simulink library "library_BCM"  (Simulink 8.2)
settings: Solver=ode45  StartTime=0.0  StopTime=10.0  RelTol=1e-3
undefined symbols (not defined in the file or in its folder): MPU_FOUR_CST, MPU_ONE_CST, MPU_THREE_CST, MPU_TWO_CST, MPU_ZERO_CST, NAMEOFTHEMODEL_SAMPLE_TIME_CST, slcm, TYP_MPU_REQUEST, TYP_MPU_REQUEST_2, TYP_MPU_STATUS, TYP_MPU_STATUS_2
libraries: Renault_Library x50, simulink x8, library_BCM x7
(part 3 of 3)

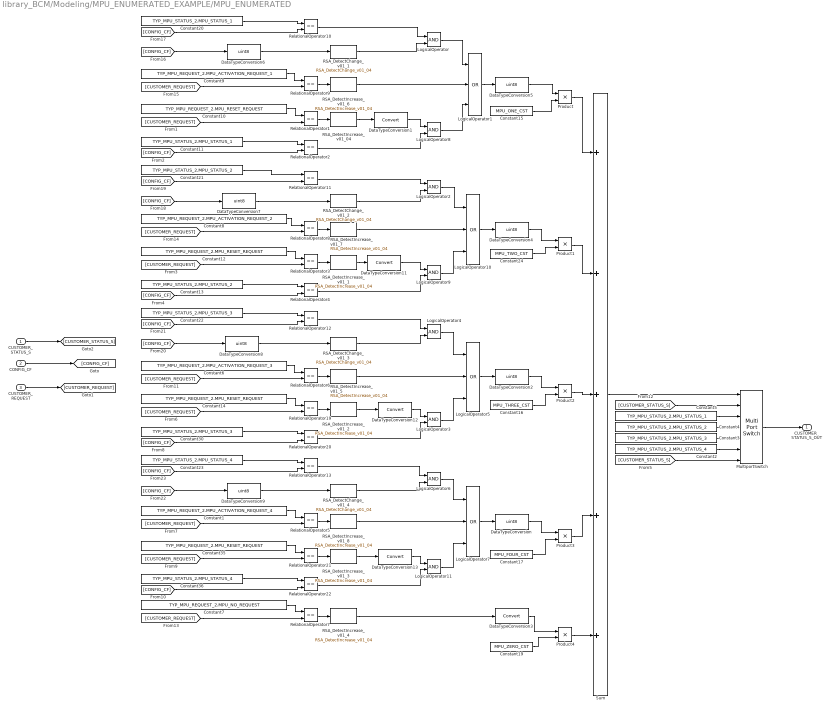
== system library_BCM/Modeling/MPU_ENUMERATED_EXAMPLE/MPU_ENUMERATED ==
  CUSTOMER_STATUS_S : Inport
      settings: AttributesFormatString=Type : %<OutDataTypeStr>
  CONFIG_CF : Inport  Port=2
      settings: AttributesFormatString=Type : %<OutDataTypeStr>
  CUSTOMER_REQUEST : Inport  Port=3
      settings: AttributesFormatString=Type : %<OutDataTypeStr>
  Constant1 : Constant  Value=TYP_MPU_REQUEST_2.MPU_ACTIVATION_REQUEST_4  OutDataTypeStr=Enum: TYP_MPU_REQUEST_2  SampleTime=-1
  Constant{10,12,14,35} (4 alike) : Constant  Value=TYP_MPU_REQUEST_2.MPU_RESET_REQUEST  OutDataTypeStr=Enum: TYP_MPU_REQUEST_2  SampleTime=-1
  Constant11 : Constant  Value=TYP_MPU_STATUS_2.MPU_STATUS_1  OutDataTypeStr=Enum: TYP_MPU_STATUS_2  SampleTime=-1
  Constant13 : Constant  Value=TYP_MPU_STATUS_2.MPU_STATUS_2  OutDataTypeStr=Enum: TYP_MPU_STATUS_2  SampleTime=-1
  Constant15 : Constant  Value=MPU_ONE_CST  OutDataTypeStr=uint8  SampleTime=-1
  Constant16 : Constant  Value=MPU_THREE_CST  OutDataTypeStr=uint8  SampleTime=-1
  Constant17 : Constant  Value=MPU_FOUR_CST  OutDataTypeStr=uint8  SampleTime=-1
  Constant19 : Constant  Value=MPU_ZERO_CST  OutDataTypeStr=uint8  SampleTime=-1
  Constant2 : Constant  Value=TYP_MPU_STATUS_2.MPU_STATUS_4  OutDataTypeStr=Enum: TYP_MPU_STATUS_2  SampleTime=-1
  Constant20 : Constant  Value=TYP_MPU_STATUS_2.MPU_STATUS_1  OutDataTypeStr=Enum: TYP_MPU_STATUS_2  SampleTime=-1
  Constant21 : Constant  Value=TYP_MPU_STATUS_2.MPU_STATUS_2  OutDataTypeStr=Enum: TYP_MPU_STATUS_2  SampleTime=-1
  Constant22 : Constant  Value=TYP_MPU_STATUS_2.MPU_STATUS_3  OutDataTypeStr=Enum: TYP_MPU_STATUS_2  SampleTime=-1
  Constant23 : Constant  Value=TYP_MPU_STATUS_2.MPU_STATUS_4  OutDataTypeStr=Enum: TYP_MPU_STATUS_2  SampleTime=-1
  Constant24 : Constant  Value=MPU_TWO_CST  OutDataTypeStr=uint8  SampleTime=-1
  Constant3 : Constant  Value=TYP_MPU_STATUS_2.MPU_STATUS_3  OutDataTypeStr=Enum: TYP_MPU_STATUS_2  SampleTime=-1
  Constant30 : Constant  Value=TYP_MPU_STATUS_2.MPU_STATUS_3  OutDataTypeStr=Enum: TYP_MPU_STATUS_2  SampleTime=-1
  Constant36 : Constant  Value=TYP_MPU_STATUS_2.MPU_STATUS_4  OutDataTypeStr=Enum: TYP_MPU_STATUS_2  SampleTime=-1
  Constant4 : Constant  Value=TYP_MPU_STATUS_2.MPU_STATUS_2  OutDataTypeStr=Enum: TYP_MPU_STATUS_2  SampleTime=-1
  Constant5 : Constant  Value=TYP_MPU_STATUS_2.MPU_STATUS_1  OutDataTypeStr=Enum: TYP_MPU_STATUS_2  SampleTime=-1
  Constant6 : Constant  Value=TYP_MPU_REQUEST_2.MPU_ACTIVATION_REQUEST_3  OutDataTypeStr=Enum: TYP_MPU_REQUEST_2  SampleTime=-1
  Constant7 : Constant  Value=TYP_MPU_REQUEST_2.MPU_NO_REQUEST  OutDataTypeStr=Enum: TYP_MPU_REQUEST_2  SampleTime=-1
  Constant8 : Constant  Value=TYP_MPU_REQUEST_2.MPU_ACTIVATION_REQUEST_2  OutDataTypeStr=Enum: TYP_MPU_REQUEST_2  SampleTime=-1
  Constant9 : Constant  Value=TYP_MPU_REQUEST_2.MPU_ACTIVATION_REQUEST_1  OutDataTypeStr=Enum: TYP_MPU_REQUEST_2  SampleTime=-1
  DataTypeConversion{,2,4..9} (8 alike) : DataTypeConversion  OutDataTypeStr=uint8  RndMeth=Zero
      settings: AttributesFormatString=Saturation:%<SaturateOnIntegerOverflow>
  DataTypeConversion{1,3,11..13} (5 alike) : DataTypeConversion  RndMeth=Zero
      settings: AttributesFormatString=Saturation:%<SaturateOnIntegerOverflow>
  LogicalOperator{,2..4,6,8..9,11} (8 alike) : Logic  OutDataTypeStr=boolean
  LogicalOperator{1,5,7,10} (4 alike) : Logic  Operator=OR  Inputs=3  OutDataTypeStr=boolean
  MultiportSwitch : MultiPortSwitch  DataPortOrder=Zero-based contiguous  Inputs=6  RndMeth=Zero  InputSameDT=on
  Product{,1..4} (5 alike) : Product  OutDataTypeStr=Inherit: Inherit via back propagation  RndMeth=Zero
  RSA_DetectChange_v01_{1..4} (4 alike) : Renault_Library/Complex blocks/Logic & Bit Operations/RSA_DetectChange_v01_04  Tag=[LIB]  chkini=off  vinit=0
      settings: AttributesFormatString=%<MaskType> : Ver : 01.04\nCompare the Input with Initial Value = %<chkini>\nInitial Value : = %<vinit>
  RSA_DetectIncrease_v01_04 : Renault_Library/Complex blocks/Logic & Bit Operations/RSA_DetectIncrease_v01_04  Tag=[LIB]  chkini=off  vinit=false
      settings: AttributesFormatString=%<MaskType> : Ver : 01.04\nCompare the Input with Initial Value = %<chkini>\nInitial Value : = %<vinit>
  RSA_DetectIncrease_v01_{1..8} (8 alike) : Renault_Library/Complex blocks/Logic & Bit Operations/RSA_DetectIncrease_v01_04  Tag=[LIB]  chkini=off  vinit=false
      settings: AttributesFormatString=%<MaskType> : Ver : 01.04\nCompare the Input with Initial Value = %<chkini>\nInitial Value : = %<vinit>
  RelationalOperator{1..13,19..22} (17 alike) : RelationalOperator  Operator===  OutDataTypeStr=boolean  InputSameDT=on
  Sum : Sum  Inputs=+++++  OutDataTypeStr=Inherit: Inherit via back propagation  RndMeth=Zero  InputSameDT=on
      settings: AttributesFormatString=Saturation:%<SaturateOnIntegerOverflow>
  CUSTOMER_STATUS_S_OUT : Outport
      settings: AttributesFormatString=Init :%<InitialOutput>
  wires:
  RelationalOperator5/1 -> RSA_DetectIncrease_v01_8/1
  LogicalOperator6/1 -> LogicalOperator7/1
  RelationalOperator13/1 -> LogicalOperator6/1
  RSA_DetectChange_v01_4/1 -> LogicalOperator6/2
  Constant23/1 -> RelationalOperator13/1
  [CONFIG_CF] -> RelationalOperator13/2
  [CONFIG_CF] -> DataTypeConversion9/1
  DataTypeConversion9/1 -> RSA_DetectChange_v01_4/1
  RelationalOperator6/1 -> RSA_DetectIncrease_v01_5/1
  LogicalOperator5/1 -> DataTypeConversion2/1
  LogicalOperator4/1 -> LogicalOperator5/1
  RelationalOperator12/1 -> LogicalOperator4/1
  RSA_DetectChange_v01_3/1 -> LogicalOperator4/2
  Constant22/1 -> RelationalOperator12/1
  [CONFIG_CF] -> RelationalOperator12/2
  [CONFIG_CF] -> DataTypeConversion8/1
  DataTypeConversion8/1 -> RSA_DetectChange_v01_3/1
  RelationalOperator8/1 -> RSA_DetectIncrease_v01_7/1
  LogicalOperator2/1 -> LogicalOperator10/1
  RelationalOperator11/1 -> LogicalOperator2/1
  RSA_DetectChange_v01_2/1 -> LogicalOperator2/2
  Constant21/1 -> RelationalOperator11/1
  [CONFIG_CF] -> RelationalOperator11/2
  [CONFIG_CF] -> DataTypeConversion7/1
  DataTypeConversion7/1 -> RSA_DetectChange_v01_2/1
  LogicalOperator1/1 -> DataTypeConversion5/1
  RelationalOperator9/1 -> RSA_DetectIncrease_v01_6/1
  LogicalOperator/1 -> LogicalOperator1/1
  RelationalOperator10/1 -> LogicalOperator/1
  RSA_DetectChange_v01_1/1 -> LogicalOperator/2
  Constant20/1 -> RelationalOperator10/1
  [CONFIG_CF] -> RelationalOperator10/2
  [CONFIG_CF] -> DataTypeConversion6/1
  DataTypeConversion6/1 -> RSA_DetectChange_v01_1/1
  Constant19/1 -> Product4/2
  Constant17/1 -> Product3/2
  Constant16/1 -> Product2/2
  Constant24/1 -> Product1/2
  Constant15/1 -> Product/2
  Product/1 -> Sum/1
  Product1/1 -> Sum/2
  Product2/1 -> Sum/3
  Product3/1 -> Sum/4
  Product4/1 -> Sum/5
  DataTypeConversion5/1 -> Product/1
  Constant9/1 -> RelationalOperator9/1
  [CUSTOMER_REQUEST] -> RelationalOperator9/2
  DataTypeConversion4/1 -> Product1/1
  Constant8/1 -> RelationalOperator8/1
  [CUSTOMER_REQUEST] -> RelationalOperator8/2
  DataTypeConversion3/1 -> Product4/1
  Constant7/1 -> RelationalOperator7/1
  [CUSTOMER_REQUEST] -> RelationalOperator7/2
  DataTypeConversion2/1 -> Product2/1
  DataTypeConversion/1 -> Product3/1
  Sum/1 -> MultiportSwitch/1
  Constant6/1 -> RelationalOperator6/1
  [CUSTOMER_REQUEST] -> RelationalOperator6/2
  Constant1/1 -> RelationalOperator5/1
  [CUSTOMER_REQUEST] -> RelationalOperator5/2
  [CUSTOMER_STATUS_S] -> MultiportSwitch/7
  MultiportSwitch/1 -> CUSTOMER_STATUS_S_OUT/1
  CONFIG_CF/1 -> [CONFIG_CF]
  CUSTOMER_REQUEST/1 -> [CUSTOMER_REQUEST]
  CUSTOMER_STATUS_S/1 -> [CUSTOMER_STATUS_S]
  RelationalOperator7/1 -> RSA_DetectIncrease_v01_4/1
  RelationalOperator1/1 -> RSA_DetectIncrease_v01_04/1
  Constant10/1 -> RelationalOperator1/1
  [CUSTOMER_REQUEST] -> RelationalOperator1/2
  RSA_DetectIncrease_v01_04/1 -> DataTypeConversion1/1
  RelationalOperator2/1 -> LogicalOperator8/2
  Constant11/1 -> RelationalOperator2/1
  [CONFIG_CF] -> RelationalOperator2/2
  DataTypeConversion1/1 -> LogicalOperator8/1
  LogicalOperator8/1 -> LogicalOperator1/3
  RelationalOperator3/1 -> RSA_DetectIncrease_v01_1/1
  Constant12/1 -> RelationalOperator3/1
  [CUSTOMER_REQUEST] -> RelationalOperator3/2
  RSA_DetectIncrease_v01_1/1 -> DataTypeConversion11/1
  RelationalOperator4/1 -> LogicalOperator9/2
  Constant13/1 -> RelationalOperator4/1
  [CONFIG_CF] -> RelationalOperator4/2
  DataTypeConversion11/1 -> LogicalOperator9/1
  LogicalOperator9/1 -> LogicalOperator10/3
  LogicalOperator10/1 -> DataTypeConversion4/1
  RelationalOperator19/1 -> RSA_DetectIncrease_v01_2/1
  Constant14/1 -> RelationalOperator19/1
  [CUSTOMER_REQUEST] -> RelationalOperator19/2
  RSA_DetectIncrease_v01_2/1 -> DataTypeConversion12/1
  RelationalOperator20/1 -> LogicalOperator3/2
  Constant30/1 -> RelationalOperator20/1
  [CONFIG_CF] -> RelationalOperator20/2
  DataTypeConversion12/1 -> LogicalOperator3/1
  LogicalOperator3/1 -> LogicalOperator5/3
  RelationalOperator21/1 -> RSA_DetectIncrease_v01_3/1
  Constant35/1 -> RelationalOperator21/1
  [CUSTOMER_REQUEST] -> RelationalOperator21/2
  RSA_DetectIncrease_v01_3/1 -> DataTypeConversion13/1
  RelationalOperator22/1 -> LogicalOperator11/2
  Constant36/1 -> RelationalOperator22/1
  [CONFIG_CF] -> RelationalOperator22/2
  DataTypeConversion13/1 -> LogicalOperator11/1
  LogicalOperator7/1 -> DataTypeConversion/1
  LogicalOperator11/1 -> LogicalOperator7/3
  RSA_DetectIncrease_v01_4/1 -> DataTypeConversion3/1
  RSA_DetectIncrease_v01_5/1 -> LogicalOperator5/2
  RSA_DetectIncrease_v01_6/1 -> LogicalOperator1/2
  RSA_DetectIncrease_v01_7/1 -> LogicalOperator10/2
  RSA_DetectIncrease_v01_8/1 -> LogicalOperator7/2
  [CUSTOMER_STATUS_S] -> MultiportSwitch/2
  Constant2/1 -> MultiportSwitch/6
  Constant5/1 -> MultiportSwitch/3
  Constant3/1 -> MultiportSwitch/5
  Constant4/1 -> MultiportSwitch/4

== system library_BCM/Validation/EEPROM/DataStoreRead ==
  Data Store Read : DataStoreRead  DataStoreName=EEPROM_S
  EEPROM_S_N : Outport
  wires:
  Data Store Read/1 -> EEPROM_S_N/1

== system library_BCM/Validation/EEPROM/DataStoreWrite ==
  EEPROM_S : Inport
  EEPROM_S_OUT : Inport  Port=2
  ECU_RESET : Inport  Port=3
  Detect Change : simulink/Logic and Bit Operations/Detect Change  vinit=0  InputProcessing=Inherited  OutDataTypeStr=boolean
  Detect Change2 : simulink/Logic and Bit Operations/Detect Change  vinit=0  InputProcessing=Inherited  OutDataTypeStr=boolean
  Detect Change4 : simulink/Logic and Bit Operations/Detect Change  vinit=0  InputProcessing=Inherited  OutDataTypeStr=boolean
  Logical Operator : Logic  AllPortsSameDT=off  OutDataTypeStr=boolean
  Logical Operator1 : Logic  Operator=NOT  AllPortsSameDT=off  OutDataTypeStr=boolean
  Subsystem : Subsystem
  Switch : Switch  Criteria=u2 ~= 0
  Switch1 : Switch  Criteria=u2 ~= 0
  Switch4 : Switch  Criteria=u2 ~= 0
  Unit Delay : UnitDelay  SampleTime=-1
  wires:
  EEPROM_S/1 -> Detect Change/1, Switch/1
  Detect Change/1 -> Switch/2
  Detect Change2/1 -> Logical Operator/1
  Logical Operator/1 -> Switch4/2
  Switch4/1 -> Switch1/3, Switch/3
  Switch/1 -> Switch1/1, Subsystem/1(In), Detect Change4/1
  Unit Delay/1 -> Switch4/3
  EEPROM_S_OUT/1 -> Detect Change2/1, Switch4/1
  Detect Change4/1 -> Subsystem/Enable
  ECU_RESET/1 -> [RESET], Logical Operator/2
  Logical Operator1/1 -> Switch1/2
  [RESET] -> Logical Operator1/1
  Switch1/1 -> Unit Delay/1

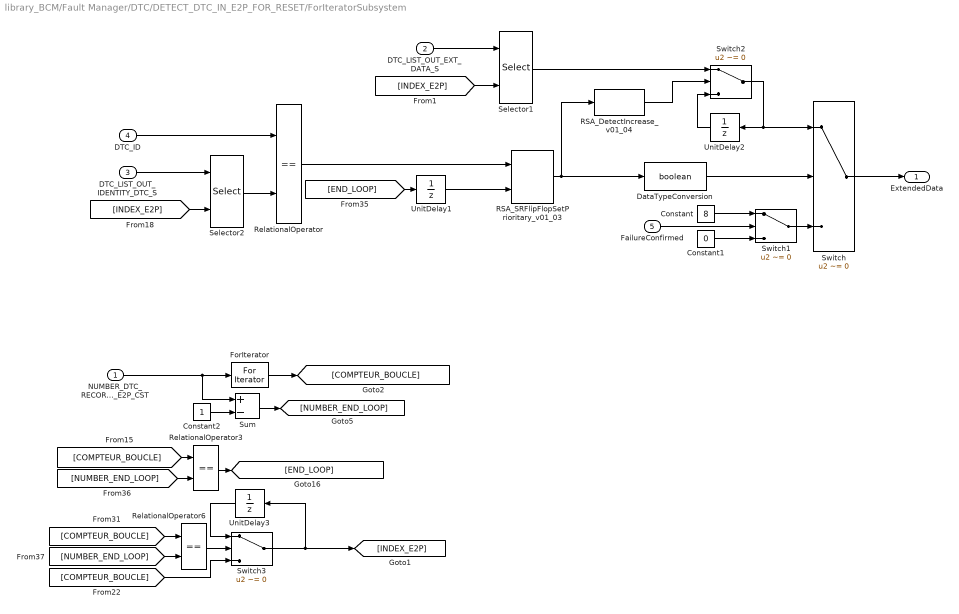
== system library_BCM/Fault Manager/DTC/DETECT_DTC_IN_E2P_FOR_RESET/ForIteratorSubsystem ==
  NUMBER_DTC_RECORD_IN_E2P_CST : Inport  OutDataTypeStr=uint32
      settings: AttributesFormatString=Type : %<OutDataTypeStr>
  DTC_LIST_OUT_EXT_DATA_S : Inport  Port=2  OutDataTypeStr=uint32
      settings: AttributesFormatString=Type : %<OutDataTypeStr>
  DTC_LIST_OUT_IDENTITY_DTC_S : Inport  Port=3  OutDataTypeStr=uint32
      settings: AttributesFormatString=Type : %<OutDataTypeStr>
  DTC_ID : Inport  Port=4  OutDataTypeStr=uint32
      settings: AttributesFormatString=Type : %<OutDataTypeStr>
  FailureConfirmed : Inport  Port=5  OutDataTypeStr=boolean
      settings: AttributesFormatString=Type : %<OutDataTypeStr>
  Constant : Constant  Value=8  OutDataTypeStr=uint32  SampleTime=-1
  Constant1 : Constant  Value=0  OutDataTypeStr=uint32  SampleTime=-1
  Constant2 : Constant  OutDataTypeStr=uint32  SampleTime=-1
  DataTypeConversion : DataTypeConversion  OutDataTypeStr=boolean  RndMeth=Zero
      settings: AttributesFormatString=Saturation:%<SaturateOnIntegerOverflow>
  ForIterator : ForIterator  IterationSource=external  IndexMode=Zero-based
  RSA_DetectIncrease_v01_04 : Renault_Library/Complex blocks/Logic & Bit Operations/RSA_DetectIncrease_v01_04  Tag=[LIB]  chkini=on  vinit=0
      settings: AttributesFormatString=%<MaskType> : Ver : 01.04\nCompare the Input with Initial Value = %<chkini>\nInitial Value : = %<vinit>
  RSA_SRFlipFlopSetPrioritary_v01_03 : Renault_Library/Complex blocks/Flip-Flop/RSA_SRFlipFlopSetPrioritary_v01_03  Tag=[LIB]  init=false
      settings: AttributesFormatString=%<MaskType> : Ver : 01.03\n<init=%<init>>
  RelationalOperator : RelationalOperator  Operator===  OutDataTypeStr=boolean  InputSameDT=on
  RelationalOperator3 : RelationalOperator  Operator===  OutDataTypeStr=boolean  InputSameDT=on
  RelationalOperator6 : RelationalOperator  Operator===  OutDataTypeStr=boolean  InputSameDT=on
  Selector1 : Selector  IndexMode=Zero-based  IndexOptions=Index vector (port)  Indices=[1 3]  OutputSizes=1
  Selector2 : Selector  IndexMode=Zero-based  IndexOptions=Index vector (port)  Indices=[1 3]  OutputSizes=1
  Sum : Sum  Inputs=+-  AccumDataTypeStr=uint32  OutDataTypeStr=Inherit: Inherit via back propagation  RndMeth=Zero  InputSameDT=on
      settings: AttributesFormatString=Saturation:%<SaturateOnIntegerOverflow>
  Switch{,1..3} (4 alike) : Switch  Criteria=u2 ~= 0  RndMeth=Zero  InputSameDT=on
      settings: AttributesFormatString=Criteria=%<Criteria>
  UnitDelay1 : UnitDelay  SampleTime=-1
      settings: AttributesFormatString=IC = %<X0>
  UnitDelay2 : UnitDelay  SampleTime=-1
      settings: AttributesFormatString=IC = %<X0>
  UnitDelay3 : UnitDelay  SampleTime=-1
      settings: AttributesFormatString=IC = %<X0>
  ExtendedData : Outport  OutDataTypeStr=uint32  InitialOutput=0
      settings: CopyFcn=if exist('tl_check_ports','file'), tl_check_ports(gcbh); end  NameChangeFcn=if exist('tl_check_ports','file'), tl_check_ports(gcbh); end
  wires:
  Constant1/1 -> Switch1/3
  Constant/1 -> Switch1/1
  Switch1/1 -> Switch/3
  FailureConfirmed/1 -> Switch1/2
  Switch/1 -> ExtendedData/1
  [INDEX_E2P] -> Selector1/2
  DTC_LIST_OUT_EXT_DATA_S/1 -> Selector1/1
  Selector2/1 -> RelationalOperator/2
  [INDEX_E2P] -> Selector2/2
  NUMBER_DTC_RECORD_IN_E2P_CST/1 -> ForIterator/1, Sum/1
  ForIterator/1 -> [COMPTEUR_BOUCLE]
  DTC_LIST_OUT_IDENTITY_DTC_S/1 -> Selector2/1
  DTC_ID/1 -> RelationalOperator/1
  [NUMBER_END_LOOP] -> RelationalOperator6/2
  UnitDelay3/1 -> Switch3/1
  [COMPTEUR_BOUCLE] -> Switch3/3
  RelationalOperator6/1 -> Switch3/2
  [COMPTEUR_BOUCLE] -> RelationalOperator6/1
  Switch3/1 -> UnitDelay3/1, [INDEX_E2P]
  [NUMBER_END_LOOP] -> RelationalOperator3/2
  RelationalOperator3/1 -> [END_LOOP]
  [COMPTEUR_BOUCLE] -> RelationalOperator3/1
  Constant2/1 -> Sum/2
  Sum/1 -> [NUMBER_END_LOOP]
  RelationalOperator/1 -> RSA_SRFlipFlopSetPrioritary_v01_03/1
  RSA_SRFlipFlopSetPrioritary_v01_03/1 -> DataTypeConversion/1, RSA_DetectIncrease_v01_04/1
  UnitDelay2/1 -> Switch2/3
  RSA_DetectIncrease_v01_04/1 -> Switch2/2
  [END_LOOP] -> UnitDelay1/1
  Switch2/1 -> UnitDelay2/1, Switch/1
  Selector1/1 -> Switch2/1
  UnitDelay1/1 -> RSA_SRFlipFlopSetPrioritary_v01_03/2
  DataTypeConversion/1 -> Switch/2

== system library_BCM/Fault Manager/DTC/DETECT_DTC_IN_E2P_FOR_RESET/TO_ADD_1_CALCUL_IN_LOOP ==
  NUMBER_DTC_RECORD_IN_E2P_CST : Inport  OutDataTypeStr=uint32
      settings: AttributesFormatString=Type : %<OutDataTypeStr>
  Constant : Constant  OutDataTypeStr=Inherit: Inherit via back propagation  SampleTime=-1
  Sum : Sum  OutDataTypeStr=Inherit: Inherit via back propagation  RndMeth=Zero  InputSameDT=on
      settings: AttributesFormatString=Saturation: %<SaturateOnIntegerOverflow>
  NB_DTC_RECORD_IN_E2P_CST_EXT : Outport  OutDataTypeStr=uint32
  wires:
  NUMBER_DTC_RECORD_IN_E2P_CST/1 -> Sum/1
  Constant/1 -> Sum/2
  Sum/1 -> NB_DTC_RECORD_IN_E2P_CST_EXT/1

== system library_BCM/Fault Manager/DTC/ExtendedData_Calcul/BitwiseLogicalOperator3 ==
  u : Inport
  shift : ArithShift  BitShiftNumber=nBitShiftRight  BinPtShiftNumber=nBinPtShiftRight
  y : Outport
  wires:
  u/1 -> shift/1
  shift/1 -> y/1

== system library_BCM/Fault Manager/DTC/ExtendedData_Calcul/BitwiseLogicalOperator6 ==
  u : Inport
  shift : ArithShift  BitShiftNumber=nBitShiftRight  BinPtShiftNumber=nBinPtShiftRight
  y : Outport
  wires:
  shift/1 -> y/1
  u/1 -> shift/1

== system library_BCM/MIL Full Matlab/Scheduling/Lib_Trigger/Trigger ==
  In1 : Inport
      settings: AttributesFormatString=Type : %<OutDataTypeStr>
  RSA_Bias1 : Subsystem  Tag=[LIB]  mask(RSA_Bias){u=1, DoSatur=off}
      mask prompts: u "Bias:"; DoSatur "Saturate on integer overflow"
      mask help:
      | Add bias to input,Y = U + Bias.
      |
      | Version : 01.00
      mask init:
      | blkH = gcbh;
      | blkName = getfullname(blkH);
      mask Display: %fprintf('u + %d', u)
  RSA_Bias2 : Subsystem  Tag=[LIB]  mask(RSA_Bias){u=-1, DoSatur=off}
      mask prompts: u "Bias:"; DoSatur "Saturate on integer overflow"
      mask help:
      | Add bias to input,Y = U + Bias.
      |
      | Version : 01.00
      mask init:
      | blkH = gcbh;
      | blkName = getfullname(blkH);
      mask Display: %fprintf('u + %d', u)
  RSA_DetectChange : Renault_Library/Complex blocks/Logic & Bit Operations/RSA_DetectChange  Tag=[LIB]  vinit=0
  RSA_DivisionByZeroWithSaturation1 : Subsystem  Tag=[LIB]  mask(RSA_DivisionByZeroWithSaturation){}
      mask help:
      | The given two inputs 'In1' and 'In2' are divided and the output 'Out1' is obtained. If the 'In2' is zero then output 'Out1' retain the input 'In1'.
      |
      | Version : 01.00
      mask Display:
      | % plot([4 12],[32 40])
      | % plot([4 12],[40 32])
      | %
      | % plot([4 12],[12 12])
      | %
      | % plot([8 8],[16 16])
      | % plot([7 9],[15 15])
      | % plot([8 8],[14 14])
      | %
      | % plot([8 8],[10 10])
      | % plot([7 9],[9 9])
      | % plot([8 8],[8 8])
  UnitDelay2 : UnitDelay  SampleTime=-1
  Out1 : Outport
      settings: AttributesFormatString=Type : %<OutDataTypeStr>\nInit :%<InitialOutput>
  wires:
  RSA_Bias1/1(Out1) -> UnitDelay2/1, RSA_Bias2/1(In1)
  UnitDelay2/1 -> RSA_Bias1/1(In1)
  RSA_Bias2/1(Out1) -> RSA_DivisionByZeroWithSaturation1/1(In1)
  RSA_DivisionByZeroWithSaturation1/1(Out1) -> RSA_DetectChange/1
  RSA_DetectChange/1 -> Out1/1
  In1/1 -> RSA_DivisionByZeroWithSaturation1/2(In2)

== system library_BCM/MIL Full Matlab/Scheduling0/Lib_Trigger/Trigger ==
  In1 : Inport
      settings: AttributesFormatString=Type : %<OutDataTypeStr>
  RSA_Bias1 : Subsystem  Tag=[LIB]  mask(RSA_Bias){u=1, DoSatur=off}
      mask prompts: u "Bias:"; DoSatur "Saturate on integer overflow"
      mask help:
      | Add bias to input,Y = U + Bias.
      |
      | Version : 01.00
      mask init:
      | blkH = gcbh;
      | blkName = getfullname(blkH);
      mask Display: %fprintf('u + %d', u)
  RSA_Bias2 : Subsystem  Tag=[LIB]  mask(RSA_Bias){u=-1, DoSatur=off}
      mask prompts: u "Bias:"; DoSatur "Saturate on integer overflow"
      mask help:
      | Add bias to input,Y = U + Bias.
      |
      | Version : 01.00
      mask init:
      | blkH = gcbh;
      | blkName = getfullname(blkH);
      mask Display: %fprintf('u + %d', u)
  RSA_DetectChange : Renault_Library/Complex blocks/Logic & Bit Operations/RSA_DetectChange  Tag=[LIB]  vinit=0
  RSA_DivisionByZeroWithSaturation1 : Subsystem  Tag=[LIB]  mask(RSA_DivisionByZeroWithSaturation){}
      mask help:
      | The given two inputs 'In1' and 'In2' are divided and the output 'Out1' is obtained. If the 'In2' is zero then output 'Out1' retain the input 'In1'.
      |
      | Version : 01.00
      mask Display:
      | % plot([4 12],[32 40])
      | % plot([4 12],[40 32])
      | %
      | % plot([4 12],[12 12])
      | %
      | % plot([8 8],[16 16])
      | % plot([7 9],[15 15])
      | % plot([8 8],[14 14])
      | %
      | % plot([8 8],[10 10])
      | % plot([7 9],[9 9])
      | % plot([8 8],[8 8])
  UnitDelay2 : UnitDelay  SampleTime=-1
  Out1 : Outport
      settings: AttributesFormatString=Type : %<OutDataTypeStr>\nInit :%<InitialOutput>
  wires:
  In1/1 -> RSA_DivisionByZeroWithSaturation1/2(In2)
  RSA_DetectChange/1 -> Out1/1
  RSA_DivisionByZeroWithSaturation1/1(Out1) -> RSA_DetectChange/1
  RSA_Bias2/1(Out1) -> RSA_DivisionByZeroWithSaturation1/1(In1)
  UnitDelay2/1 -> RSA_Bias1/1(In1)
  RSA_Bias1/1(Out1) -> RSA_Bias2/1(In1), UnitDelay2/1

== system library_BCM/Validation/EEPROM/DataStoreWrite/Subsystem ==
  In : Inport
  Enable : EnablePort  StatesWhenEnabling=reset
  Data Store Write : DataStoreWrite  DataStoreName=EEPROM_S
  wires:
  In/1 -> Data Store Write/1

== system library_BCM/MIL Full Matlab/Scheduling/Lib_Trigger/Trigger/RSA_Bias1 ==
  In1 : Inport
      settings: AttributesFormatString=Type : %<OutDataType>\nScaling : %<OutScaling>
  Add : Sum  OutDataTypeStr=Inherit: Inherit via back propagation  RndMeth=Zero  InputSameDT=on
  Constant1 : Constant  Value=u  OutDataTypeStr=Inherit: Inherit via back propagation  SampleTime=-1
  Out1 : Outport
      settings: AttributesFormatString=Type : %<OutDataType>\nScaling : %<OutScaling>\nInit :%<InitialOutput>
  wires:
  Constant1/1 -> Add/2
  In1/1 -> Add/1
  Add/1 -> Out1/1

== system library_BCM/MIL Full Matlab/Scheduling/Lib_Trigger/Trigger/RSA_Bias2 ==
  In1 : Inport
      settings: AttributesFormatString=Type : %<OutDataType>\nScaling : %<OutScaling>
  Add : Sum  OutDataTypeStr=Inherit: Inherit via back propagation  RndMeth=Zero  InputSameDT=on
  Constant1 : Constant  Value=u  OutDataTypeStr=Inherit: Inherit via back propagation  SampleTime=-1
  Out1 : Outport
      settings: AttributesFormatString=Type : %<OutDataType>\nScaling : %<OutScaling>\nInit :%<InitialOutput>
  wires:
  Add/1 -> Out1/1
  In1/1 -> Add/1
  Constant1/1 -> Add/2

== system library_BCM/MIL Full Matlab/Scheduling/Lib_Trigger/Trigger/RSA_DivisionByZeroWithSaturation1 ==
  In1 : Inport
      settings: AttributesFormatString=Type : %<OutDataType>\nScaling : %<OutScaling>
  In2 : Inport  Port=2
      settings: AttributesFormatString=Type : %<OutDataType>\nScaling : %<OutScaling>
  Product2 : Product  Inputs=*/  OutDataTypeStr=Inherit: Inherit via back propagation  RndMeth=Zero  InputSameDT=on
  RSA_CompareToZero : Subsystem  Tag=[LIB]  mask(RSA_CompareToZero){relop===, LogicOutDataTypeMode=boolean, ZeroCross=on}
      mask prompts: relop "Operator:"; LogicOutDataTypeMode "Output data type mode:"; ZeroCross "Enable zero-crossing detection"
      mask help:
      | Output of the block will be zero when the signal is less than or equal to zero otherwise it will be one.
      |
      | Version : 01.00
      mask init:
      | blkName = gcb;
      mask TypeOptions relop: == | ~= | < | <= | >= | >
      mask TypeOptions LogicOutDataTypeMode: uint8 | boolean
      mask Display: disp([relop,' 0'])
  Switch1 : Switch  Criteria=u2 ~= 0  RndMeth=Zero  SaturateOnIntegerOverflow=on  InputSameDT=on
  const1 : Constant  OutDataTypeStr=Inherit: Inherit via back propagation  SampleTime=-1
  Out1 : Outport
      settings: AttributesFormatString=Type : %<OutDataType>\nScaling : %<OutScaling>\nInit :%<InitialOutput>
  wires:
  In1/1 -> Product2/1
  Product2/1 -> Out1/1
  const1/1 -> Switch1/1
  Switch1/1 -> Product2/2
  RSA_CompareToZero/1(y) -> Switch1/2
  In2/1 -> Switch1/3, RSA_CompareToZero/1(u)

== system library_BCM/MIL Full Matlab/Scheduling0/Lib_Trigger/Trigger/RSA_Bias1 ==
  In1 : Inport
      settings: AttributesFormatString=Type : %<OutDataType>\nScaling : %<OutScaling>
  Add : Sum  OutDataTypeStr=Inherit: Inherit via back propagation  RndMeth=Zero  InputSameDT=on
  Constant1 : Constant  Value=u  OutDataTypeStr=Inherit: Inherit via back propagation  SampleTime=-1
  Out1 : Outport
      settings: AttributesFormatString=Type : %<OutDataType>\nScaling : %<OutScaling>\nInit :%<InitialOutput>
  wires:
  Add/1 -> Out1/1
  In1/1 -> Add/1
  Constant1/1 -> Add/2

== system library_BCM/MIL Full Matlab/Scheduling0/Lib_Trigger/Trigger/RSA_Bias2 ==
  In1 : Inport
      settings: AttributesFormatString=Type : %<OutDataType>\nScaling : %<OutScaling>
  Add : Sum  OutDataTypeStr=Inherit: Inherit via back propagation  RndMeth=Zero  InputSameDT=on
  Constant1 : Constant  Value=u  OutDataTypeStr=Inherit: Inherit via back propagation  SampleTime=-1
  Out1 : Outport
      settings: AttributesFormatString=Type : %<OutDataType>\nScaling : %<OutScaling>\nInit :%<InitialOutput>
  wires:
  Constant1/1 -> Add/2
  In1/1 -> Add/1
  Add/1 -> Out1/1

== system library_BCM/MIL Full Matlab/Scheduling0/Lib_Trigger/Trigger/RSA_DivisionByZeroWithSaturation1 ==
  In1 : Inport
      settings: AttributesFormatString=Type : %<OutDataType>\nScaling : %<OutScaling>
  In2 : Inport  Port=2
      settings: AttributesFormatString=Type : %<OutDataType>\nScaling : %<OutScaling>
  Product2 : Product  Inputs=*/  OutDataTypeStr=Inherit: Inherit via back propagation  RndMeth=Zero  InputSameDT=on
  RSA_CompareToZero : Subsystem  Tag=[LIB]  mask(RSA_CompareToZero){relop===, LogicOutDataTypeMode=boolean, ZeroCross=on}
      mask prompts: relop "Operator:"; LogicOutDataTypeMode "Output data type mode:"; ZeroCross "Enable zero-crossing detection"
      mask help:
      | Output of the block will be zero when the signal is less than or equal to zero otherwise it will be one.
      |
      | Version : 01.00
      mask init:
      | blkName = gcb;
      mask TypeOptions relop: == | ~= | < | <= | >= | >
      mask TypeOptions LogicOutDataTypeMode: uint8 | boolean
      mask Display: disp([relop,' 0'])
  Switch1 : Switch  Criteria=u2 ~= 0  RndMeth=Zero  SaturateOnIntegerOverflow=on  InputSameDT=on
  const1 : Constant  OutDataTypeStr=Inherit: Inherit via back propagation  SampleTime=-1
  Out1 : Outport
      settings: AttributesFormatString=Type : %<OutDataType>\nScaling : %<OutScaling>\nInit :%<InitialOutput>
  wires:
  In2/1 -> RSA_CompareToZero/1(u), Switch1/3
  RSA_CompareToZero/1(y) -> Switch1/2
  Switch1/1 -> Product2/2
  const1/1 -> Switch1/1
  Product2/1 -> Out1/1
  In1/1 -> Product2/1

== system library_BCM/MIL Full Matlab/Scheduling/Lib_Trigger/Trigger/RSA_DivisionByZeroWithSaturation1/RSA_CompareToZero ==
  u : Inport
      settings: AttributesFormatString=Type : %<OutDataType>\nScaling : %<OutScaling>
  Compare : RelationalOperator  Operator===  OutDataTypeStr=boolean  InputSameDT=on
  Constant : Constant  DisableCoverage=on  Value=0  OutDataTypeStr=Inherit: Inherit via back propagation  SampleTime=-1  PreserveConstantTs=on
  y : Outport
      settings: AttributesFormatString=Type : %<OutDataType>\nScaling : %<OutScaling>\nInit :%<InitialOutput>
  wires:
  Constant/1 -> Compare/2
  u/1 -> Compare/1
  Compare/1 -> y/1

== system library_BCM/MIL Full Matlab/Scheduling0/Lib_Trigger/Trigger/RSA_DivisionByZeroWithSaturation1/RSA_CompareToZero ==
  u : Inport
      settings: AttributesFormatString=Type : %<OutDataType>\nScaling : %<OutScaling>
  Compare : RelationalOperator  Operator===  OutDataTypeStr=boolean  InputSameDT=on
  Constant : Constant  DisableCoverage=on  Value=0  OutDataTypeStr=Inherit: Inherit via back propagation  SampleTime=-1  PreserveConstantTs=on
  y : Outport
      settings: AttributesFormatString=Type : %<OutDataType>\nScaling : %<OutScaling>\nInit :%<InitialOutput>
  wires:
  Compare/1 -> y/1
  u/1 -> Compare/1
  Constant/1 -> Compare/2

== stateflow chart Validation/EEPROM_OLD/Chart ==
  state A
  (default) -> A : {
      | x=1;
      | }
  A -> A [order 1] : [hasChanged(WRITE)]
      | {
      | x=2;
      | }
  A -> A [order 2] : [hasChanged(READ)]
      | {
      | x=1;
      | }
  data: READ input double; WRITE input double; x output double

== stateflow chart Fault Manager/EEPROM_SNAPSHOT/EEPROM_FCT/EEPROM_chart ==
  note: /*effacement de l'indice du DTC ecrit */
  note: /*mise à jour SNAPSHOT*/
  note: /*i_IDENTITYFULL = 0 ==> init
      | i_IDENTITYFULL = 1==> new DTC already saved in EEPROM
      | i_IDENTITYFULL = 2 ==> new DTC is not saved in EEPROM and empty case is available
      | i_IDENTITYFULL =3 ==> new DTC is not saved in EEPROM and empty case is not available*/
  (default) -> (junction 50) : /* boucle recupération index TCONF montés */
      | {i_RAM=0;
      | i_TCONF=0;
      | DTC_LIST_OUT_OCCUR_CNT_S_INT=DTC_LIST_OUT_OCCUR_CNT_S;
      | DTC_LIST_OUT_EXT_DATA_S_INT=DTC_LIST_OUT_EXT_DATA_S;
      | DTC_LIST_OUT_IDENTITY_DTC_S_INT=DTC_LIST_OUT_IDENTITY_DTC_S;
      | DTC_LIST_OUT_SNAPSHOT_S_INT=DTC_LIST_OUT_SNAPSHOT_S;
      | NB_PRESENT_DTC_S_INT=NB_PRESENT_DTC_S;
      | NUMBER_TCONF_TO_UPDATE=NUMBER_TCONF_UP;}
  (junction 51) -> (junction 50) [order 1] : [i_RAM<NUMBER_DTC_RECORD_IN_RAM]
  (junction 50) -> (junction 51) [order 1] : [TCONF_CHANGED[i_RAM]==1]
      | {TCONF_CHANGED_SIMPLIFIED[i_TCONF]=i_RAM;
      | i_TCONF=i_TCONF+1;
      | i_RAM=i_RAM+1;}
  (junction 50) -> (junction 51) [order 2] : {i_RAM=i_RAM+1;}
  (junction 51) -> (junction 52) [order 2] : /* boucle vérification déjà présent */
      | {i_TCONF=0;
      | i_SNAPSHOT=0;
      | i_EEPROM=0;
      | i_IDENTITYFULL=0;}
  (junction 53) -> (junction 54) [order 1] : [(((STATUS_TABLE[TCONF_CHANGED_SIMPLIFIED[i_TCONF]])&0xFFFFFFF0)>>4)!=0x0FFFFFFF]
      | {
      | DTC_LIST_OUT_EXT_DATA_S_INT[i_EEPROM]=STATUS_TABLE[TCONF_CHANGED_SIMPLIFIED[i_TCONF]];
      | }
  (junction 52) -> (junction 53) [order 2] : [DTC_ID[TCONF_CHANGED_SIMPLIFIED[i_TCONF]]==DTC_LIST_OUT_IDENTITY_DTC_S_INT[i_EEPROM]]
      | {
      | DTC_LIST_OUT_IDENTITY_DTC_S_INT[i_EEPROM]=DTC_ID[TCONF_CHANGED_SIMPLIFIED[i_TCONF]];
      | i_TCONF_TEMP=i_TCONF;
      | NUMBER_TCONF_TO_UPDATE=NUMBER_TCONF_TO_UPDATE-1;
      | i_IDENTITYFULL=1;
      | }
  (junction 52) -> (junction 61) [order 1] : /*pas de DTC à cet index */
      | [DTC_ID[TCONF_CHANGED_SIMPLIFIED[i_TCONF]]==0]
  (junction 53) -> (junction 54) [order 2]
  (junction 54) -> (junction 60) [order 1] : [DTC_LIST_OUT_OCCUR_CNT_S_INT[i_EEPROM]==255]
  (junction 56) -> (junction 52) [order 1] : [i_TCONF<NUMBER_TCONF_TO_UPDATE]
  (junction 52) -> (junction 57) [order 3] : {i_EEPROM=i_EEPROM+1;}
  (junction 54) -> (junction 60) [order 2] : {DTC_LIST_OUT_OCCUR_CNT_S_INT[i_EEPROM]=DTC_LIST_OUT_OCCUR_CNT_S_INT[i_EEPROM]+1;}
  (junction 55) -> (junction 58) [order 1] : [i_TCONF_TEMP<NUMBER_TCONF_TO_UPDATE-1]
      | {i_TCONF_TEMP=i_TCONF_TEMP+1;}
  (junction 59) -> (junction 60) [order 1] : [i_SNAPSHOT<SNAPSHOT_MAX_LENGHT-1]
      | {i_SNAPSHOT=i_SNAPSHOT+1;}
  (junction 55) -> (junction 57) [order 3] : {i_EEPROM=0;}
  (junction 57) -> (junction 56) [order 2] : {i_TCONF=i_TCONF+1;
      | i_EEPROM=0;}
  (junction 59) -> (junction 58) [order 2] : [i_IDENTITYFULL!=3]{i_SNAPSHOT=0;}
  (junction 56) -> (junction 61) [order 2]
  (junction 60) -> (junction 59) [order 3] : {DTC_LIST_OUT_SNAPSHOT_S_INT[i_SNAPSHOT][i_EEPROM]=SNAPSHOT_TABLE[i_SNAPSHOT][TABLE_DTC_SNAPSHOT_NUMBER_CONV[TCONF_CHANGED_SIMPLIFIED[i_TCONF]]];}
  (junction 58) -> (junction 55) : {TCONF_CHANGED_SIMPLIFIED[i_TCONF_TEMP]=TCONF_CHANGED_SIMPLIFIED[i_TCONF_TEMP+1];}
  (junction 55) -> (junction 63) [order 2] : [i_IDENTITYFULL==2]
  (junction 60) -> (junction 59) [order 2] : [i_IDENTITYFULL==2]{DTC_LIST_OUT_SNAPSHOT_S_INT[i_SNAPSHOT][NB_PRESENT_DTC_S_INT-1]=SNAPSHOT_TABLE[i_SNAPSHOT][TABLE_DTC_SNAPSHOT_NUMBER_CONV[TCONF_CHANGED_SIMPLIFIED[i_TCONF]]];}
  (junction 59) -> (junction 66) [order 3] : {i_SNAPSHOT=0;}
  (junction 62) -> (junction 60) [order 1] : [DTC_LIST_OUT_IDENTITY_DTC_S_INT[NB_PRESENT_DTC_S_INT]==0]
      | {
      | DTC_LIST_OUT_IDENTITY_DTC_S_INT[NB_PRESENT_DTC_S_INT]=DTC_ID[TCONF_CHANGED_SIMPLIFIED[i_TCONF]];
      | DTC_LIST_OUT_EXT_DATA_S_INT[NB_PRESENT_DTC_S_INT]=STATUS_TABLE[TCONF_CHANGED_SIMPLIFIED[i_TCONF]];
      | DTC_LIST_OUT_OCCUR_CNT_S_INT[NB_PRESENT_DTC_S_INT]=1;
      | i_TCONF_TEMP=i_TCONF;
      | NUMBER_TCONF_TO_UPDATE=NUMBER_TCONF_TO_UPDATE-1;
      | i_IDENTITYFULL=2;
      | NB_PRESENT_DTC_S_INT++;
      | }
  (junction 57) -> (junction 56) [order 1] : [i_EEPROM<NUMBER_DTC_RECORD_IN_EEPROM]
  (junction 60) -> (junction 59) [order 1] : [i_IDENTITYFULL==3]{DTC_LIST_OUT_SNAPSHOT_S_INT[i_SNAPSHOT][i_DISTANCE_MINI]=SNAPSHOT_TABLE[i_SNAPSHOT][TABLE_DTC_SNAPSHOT_NUMBER_CONV[TCONF_CHANGED_SIMPLIFIED[i_TCONF]]];}
  (junction 69) -> (junction 60) [order 2] : {
      | DTC_LIST_OUT_IDENTITY_DTC_S_INT[i_DISTANCE_MINI]=DTC_ID[TCONF_CHANGED_SIMPLIFIED[i_TCONF]];
      | DTC_LIST_OUT_EXT_DATA_S_INT[i_DISTANCE_MINI]=STATUS_TABLE[TCONF_CHANGED_SIMPLIFIED[i_TCONF]];
      | DTC_LIST_OUT_OCCUR_CNT_S_INT[i_DISTANCE_MINI]=1;
      | NUMBER_TCONF_TO_UPDATE=NUMBER_TCONF_TO_UPDATE-1;
      | DISTANCE_UNAVAILABLE_FIND=false;
      | }
  (junction 61) -> (junction 65) [order 1] : [NUMBER_TCONF_TO_UPDATE==0]
  (junction 61) -> (junction 63) [order 2] : {i_TCONF=0;
      | i_EEPROM=0;
      | i_SNAPSHOT=0;}
  (junction 63) -> (junction 62) [order 2] : [NB_PRESENT_DTC_S_INT<=(NUMBER_DTC_RECORD_IN_EEPROM-1)]
  (junction 62) -> (junction 67) [order 2] : {i_TCONF=0;
      | i_EEPROM=0;
      | i_SNAPSHOT=0;}
  (junction 63) -> (junction 65) [order 1] : [NUMBER_TCONF_TO_UPDATE==0]
  (junction 63) -> (junction 67) [order 3] : {i_TCONF=0;
      | i_EEPROM=0;
      | i_SNAPSHOT=0;}
  (junction 65) -> (junction 64) : {DTC_LIST_OUT_IDENTITY_DTC_S_OUT=DTC_LIST_OUT_IDENTITY_DTC_S_INT;
      | DTC_LIST_OUT_EXT_DATA_S_OUT=DTC_LIST_OUT_EXT_DATA_S_INT;
      | DTC_LIST_OUT_SNAPSHOT_S_OUT=DTC_LIST_OUT_SNAPSHOT_S_INT;
      | DTC_LIST_OUT_OCCUR_CNT_S_OUT=DTC_LIST_OUT_OCCUR_CNT_S_INT;
      | NB_PRESENT_DTC_S_OUT=NB_PRESENT_DTC_S_INT;}
  (junction 66) -> (junction 65) [order 2]
  (junction 68) -> (junction 69) [order 1] : [((DTC_LIST_OUT_EXT_DATA_S_INT[i_EEPROM]&0xFFFFFFF0)>>4)==0x0FFFFFFF]
      | {DISTANCE_UNAVAILABLE_FIND=true;
      | i_DISTANCE_MINI=i_EEPROM;}
  (junction 68) -> (junction 69) [order 2] : [(DTC_LIST_OUT_EXT_DATA_S_INT[i_EEPROM]&0xFFFFFFF0)<DISTANCE_MINI]
      | {DISTANCE_MINI=(DTC_LIST_OUT_EXT_DATA_S_INT[i_EEPROM]&0xFFFFFFF0);
      | i_DISTANCE_MINI=i_EEPROM;}
  (junction 66) -> (junction 67) [order 1] : [NUMBER_TCONF_TO_UPDATE>0]
      | {i_TCONF=i_TCONF+1;
      | i_EEPROM=0;}
  (junction 67) -> (junction 68) : {DISTANCE_MINI=DTC_LIST_OUT_EXT_DATA_S_INT[i_EEPROM]&0xFFFFFFF0;
      | i_DISTANCE_MINI=i_EEPROM;
      | i_EEPROM=i_EEPROM;
      | i_IDENTITYFULL=3;}
  (junction 68) -> (junction 69) [order 3]
  (junction 69) -> (junction 68) [order 1] : [(i_EEPROM<NUMBER_DTC_RECORD_IN_EEPROM-1) && (DISTANCE_UNAVAILABLE_FIND==false)]
      | {i_EEPROM=i_EEPROM+1;}
  data: i_RAM local uint8; i_TCONF local uint8; NUMBER_DTC_RECORD_IN_RAM input uint8 =7; TCONF_CHANGED input double; NUMBER_TCONF_UP input double; DTC_LIST_OUT_EXT_DATA_S_OUT output uint32 size=[NUMBER_DTC_RECORD_IN_E2P_CST]; DTC_LIST_OUT_IDENTITY_DTC_S_OUT output uint32 size=[NUMBER_DTC_RECORD_IN_E2P_CST]; DTC_LIST_OUT_SNAPSHOT_S_OUT output uint8 size=[SNAPSHOT_MAX_LENGHT NUMBER_DTC_RECORD_IN_E2P_CST]; DTC_LIST_OUT_OCCUR_CNT_S_OUT output uint8 size=[NUMBER_DTC_RECORD_IN_E2P_CST]; DISTANCE_MINI local uint32; DTC_LIST_OUT_EXT_DATA_S_INT local uint32 size=[NUMBER_DTC_RECORD_IN_E2P_CST]; DTC_LIST_OUT_IDENTITY_DTC_S_INT local uint32 size=[NUMBER_DTC_RECORD_IN_E2P_CST]; DTC_LIST_OUT_OCCUR_CNT_S_INT local uint8 size=[NUMBER_DTC_RECORD_IN_E2P_CST]; DTC_LIST_OUT_SNAPSHOT_S_INT local uint8 size=[SNAPSHOT_MAX_LENGHT NUMBER_DTC_RECORD_IN_E2P_CST]; NUMBER_TCONF_TO_UPDATE local uint8; i_DISTANCE_MINI local uint8; i_EEPROM local uint8; i_TCONF_TEMP local uint8; DTC_ID input double; DTC_LIST_OUT_IDENTITY_DTC_S input double; DTC_LIST_OUT_OCCUR_CNT_S input double; NUMBER_DTC_RECORD_IN_EEPROM input uint8 =3; SNAPSHOT_TABLE input double; STATUS_TABLE input double; TABLE_DTC_SNAPSHOT_NUMBER_CONV input double; TCONF_CHANGED_SIMPLIFIED local uint8 size=[NUMBER_DTC_RECORD_IN_RAM_CST]; DTC_LIST_OUT_EXT_DATA_S input double; DTC_LIST_OUT_SNAPSHOT_S input double; i_SNAPSHOT local double; SNAPSHOT_MAX_LENGHT input double; i_IDENTITYFULL local double; NB_PRESENT_DTC_S_OUT output uint8; NB_PRESENT_DTC_S_INT local uint8 size=1; NB_PRESENT_DTC_S input double; DISTANCE_UNAVAILABLE_FIND local boolean

== stateflow chart MIL Full Matlab/Scheduler ==
  state Scheduler
    on every(1,Call): send(Sched_5ms);
    on every(2,Call): send(Sched_10ms);
    on every(3,Call): send(Sched_15ms);
    on every(4,Call): send(Sched_20ms);
    on every(6,Call): send(Sched_30ms);
    on every(8,Call): send(Sched_40ms);
    on every(10,Call): send(Sched_50ms);
    on every(20,Call): send(Sched_100ms);
    on every(30,Call): send(Sched_150ms);
    on every(40,Call): send(Sched_200ms);
  (default) -> Scheduler
  events: Sched_5ms output FUNCTION_CALL_EVENT; Sched_10ms output FUNCTION_CALL_EVENT; Sched_15ms output FUNCTION_CALL_EVENT; Sched_20ms output FUNCTION_CALL_EVENT; Sched_30ms output FUNCTION_CALL_EVENT; Sched_40ms output FUNCTION_CALL_EVENT; Sched_50ms output FUNCTION_CALL_EVENT; Sched_100ms output FUNCTION_CALL_EVENT; Call input FUNCTION_CALL_EVENT; Sched_150ms output FUNCTION_CALL_EVENT; Sched_200ms output FUNCTION_CALL_EVENT
